simulink library "LIB_TF_G_12_StepControl"  (Simulink 8.6)
settings: Solver=ode45  StartTime=0.0  StopTime=10.0  RelTol=1e-3
PreLoadFcn:
  | if exist('tl_preloadfcn','file'), tl_preloadfcn(gcs,402); end
PostLoadFcn:
  | if exist('tl_postloadfcn','file'), tl_postloadfcn(gcs,402); end
undefined symbols (not defined in the file or in its folder): ddv
libraries: tllib x2
(part 1 of 2)
CloseFcn:
  | if exist('tl_closefcn','file'), tl_closefcn(gcs); end
settings Model: TLRevision=402  Creator=cedric.sauvage  LastModifiedBy=ioan.repede

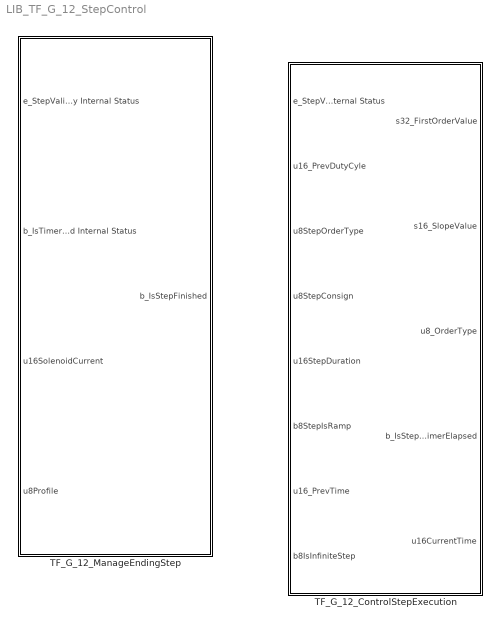
== system LIB_TF_G_12_StepControl ==
  TF_G_12_ControlStepExecution : Subsystem  TreatAsAtomicUnit=on
  TF_G_12_ManageEndingStep : Subsystem  TreatAsAtomicUnit=on

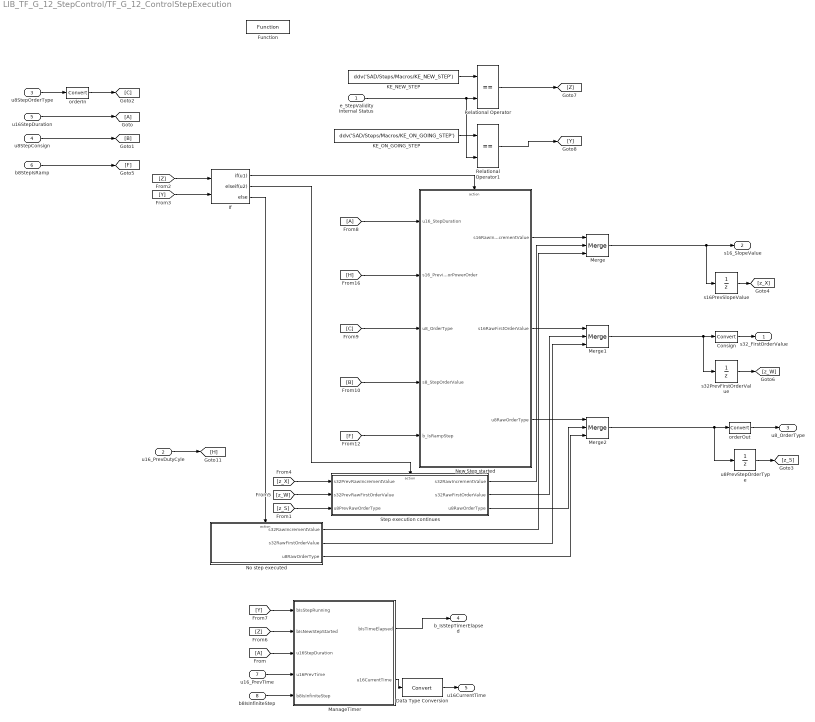
== system LIB_TF_G_12_StepControl/TF_G_12_ControlStepExecution ==
  e_StepValidity Internal Status : Inport
  u16_PrevDutyCyle : Inport  Port=2
  u8StepOrderType : Inport  Port=3
  u8StepConsign : Inport  Port=4
  u16StepDuration : Inport  Port=5
  b8StepIsRamp : Inport  Port=6
  u16_PrevTime : Inport  Port=7
  b8IsInfiniteStep : Inport  Port=8
  Consign : DataTypeConversion  mask(TL_Rescaler){data={'logdata',{'loggingmode',1},'output',{'type','UInt16'},'date',738430.45688642364}}
      settings: DeleteFcn=if exist('delete_tlblock','file')==2,delete_tlblock(gcbh);end  NameChangeFcn=if exist('rename_tlblock','file')==2,rename_tlblock(gcbh);end  OpenFcn=if exist('tl_open_blockdlg','file')==2,tl_open_blockdlg(gcbh);else,open_system(gcbh,'parameter');end
      mask Help: eval(['if exist(''tl_online_help'',''file'') == 2, tl_online_help(''Topic'',''TL_Rescaler''),else, web([''jar:file:///'',matlabroot,''/help/toolbox/simulink/help.jar!/slref/' lower(get_param(gcbh,'Blocktype')) '.html''], ''-helpbrowser''),end'])
      mask Display: plot([-0.1, 1.05, NaN, -0.1, 1.05],[.01, .01, NaN, .99, .99]);
  Data Type Conversion : DataTypeConversion
  Function : tllib/Function  RequirementInfo={'other' '..\..\..\..\Documents and Settings\cedric.sauvage\Desktop\BFE_Design.doc' '@Simulink_requirement_item_16' 'true' 'DSG_BFE_00033' '' } %GIDa_aa7399e7_4aec_40ce_b84e_da620cbb38ff  data={'stepfunctionname','M_ControlStepExecution','stepfunctionclass','STATIC_FCN','codecomment',['[COVERS: DSG_BFE_00033]'],'date',738317.69240863423}  displayString=FUNCTION
  If : If  RequirementInfo={} %GIDa_dfdbd0a4_334d_4bd1_9cca_3fcb5b10a1a1  NumInputs=2  IfExpression=u1  ElseIfExpressions=u2
  KE_NEW_STEP : Constant  Value=ddv('SAD/Steps/Macros/KE_NEW_STEP')  mask(TL_Constant){data={'output',{'variable','SAD/Steps/Macros/KE_NEW_STEP'},'date',738317.69197002309}}
      settings: CopyFcn=if exist('tl_reset_reviewflag','file')==2,tl_reset_reviewflag(gcbh);end  DeleteFcn=if exist('delete_tlblock','file')==2,delete_tlblock(gcbh);end  NameChangeFcn=if exist('rename_tlblock','file')==2,rename_tlblock(gcbh);end  OpenFcn=if exist('tl_open_blockdlg','file')==2,tl_open_blockdlg(gcbh);else,open_system(gcbh,'parameter');end
      mask Help: eval(['if exist(''tl_online_help'',''file'') == 2, tl_online_help(''Topic'',''TL_Constant''),else, web([''jar:file:///'',matlabroot,''/help/toolbox/simulink/help.jar!/slref/' lower(get_param(gcbh,'Blocktype')) '.html''], ''-helpbrowser''),end'])
      mask Display: plot([-0.05, 1.05, NaN, -0.05, 1.05],[.01, .01, NaN, .99, .99])
  KE_ON_GOING_STEP : Constant  Value=ddv('SAD/Steps/Macros/KE_ON_GOING_STEP')  mask(TL_Constant){data={'output',{'variable','SAD/Steps/Macros/KE_ON_GOING_STEP'},'date',738317.69212677085}}
      settings: CopyFcn=if exist('tl_reset_reviewflag','file')==2,tl_reset_reviewflag(gcbh);end  DeleteFcn=if exist('delete_tlblock','file')==2,delete_tlblock(gcbh);end  NameChangeFcn=if exist('rename_tlblock','file')==2,rename_tlblock(gcbh);end  OpenFcn=if exist('tl_open_blockdlg','file')==2,tl_open_blockdlg(gcbh);else,open_system(gcbh,'parameter');end
      mask Help: eval(['if exist(''tl_online_help'',''file'') == 2, tl_online_help(''Topic'',''TL_Constant''),else, web([''jar:file:///'',matlabroot,''/help/toolbox/simulink/help.jar!/slref/' lower(get_param(gcbh,'Blocktype')) '.html''], ''-helpbrowser''),end'])
      mask Display: plot([-0.05, 1.05, NaN, -0.05, 1.05],[.01, .01, NaN, .99, .99])
  ManageTimer : Subsystem  RequirementInfo={} %GIDa_1c6e116c_deb6_4c8b_9c2a_a3ed8f535171  TreatAsAtomicUnit=on
      settings: RTWFcnNameOpts=Use subsystem name
  Merge : Merge  Inputs=3  InitialOutput=0  mask(TL_Merge){data={'output',{'name','s32RawIncrementValue'},'date',735951.66799646989}}
      settings: CopyFcn=if exist('tl_reset_reviewflag','file')==2,tl_reset_reviewflag(gcbh);end  DeleteFcn=if exist('delete_tlblock','file')==2,delete_tlblock(gcbh);end  NameChangeFcn=if exist('rename_tlblock','file')==2,rename_tlblock(gcbh);end  OpenFcn=if exist('tl_open_blockdlg','file')==2,tl_open_blockdlg(gcbh);else,open_system(gcbh,'parameter');end
      mask Help: eval(['if exist(''tl_online_help'',''file'') == 2, tl_online_help(''Topic'',''TL_Merge''),else, web([''jar:file:///'',matlabroot,''/help/toolbox/simulink/help.jar!/slref/' lower(get_param(gcbh,'Blocktype')) '.html''], ''-helpbrowser''),end'])
      mask Display: plot([-0.05, 1.05, NaN, -0.05, 1.05],[.01, .01, NaN, .99, .99])
  Merge1 : Merge  Inputs=3  InitialOutput=0  mask(TL_Merge){data={'output',{'name','s32RawFirstOrderValue'},'date',735951.66799608793}}
      settings: CopyFcn=if exist('tl_reset_reviewflag','file')==2,tl_reset_reviewflag(gcbh);end  DeleteFcn=if exist('delete_tlblock','file')==2,delete_tlblock(gcbh);end  NameChangeFcn=if exist('rename_tlblock','file')==2,rename_tlblock(gcbh);end  OpenFcn=if exist('tl_open_blockdlg','file')==2,tl_open_blockdlg(gcbh);else,open_system(gcbh,'parameter');end
      mask Help: eval(['if exist(''tl_online_help'',''file'') == 2, tl_online_help(''Topic'',''TL_Merge''),else, web([''jar:file:///'',matlabroot,''/help/toolbox/simulink/help.jar!/slref/' lower(get_param(gcbh,'Blocktype')) '.html''], ''-helpbrowser''),end'])
      mask Display: plot([-0.05, 1.05, NaN, -0.05, 1.05],[.01, .01, NaN, .99, .99])
  Merge2 : Merge  RequirementInfo={} %GIDa_81538ec5_5da8_4e36_98a9_b64854f730e2  Inputs=3  InitialOutput=7  mask(TL_Merge){data={'output',{'name','u8RawOrderType'},'date',738370.40050972218}}
      settings: CopyFcn=if exist('tl_reset_reviewflag','file')==2,tl_reset_reviewflag(gcbh);end  DeleteFcn=if exist('delete_tlblock','file')==2,delete_tlblock(gcbh);end  NameChangeFcn=if exist('rename_tlblock','file')==2,rename_tlblock(gcbh);end  OpenFcn=if exist('tl_open_blockdlg','file')==2,tl_open_blockdlg(gcbh);else,open_system(gcbh,'parameter');end
      mask Help: eval(['if exist(''tl_online_help'',''file'') == 2, tl_online_help(''Topic'',''TL_Merge''),else, web([''jar:file:///'',matlabroot,''/help/toolbox/simulink/help.jar!/slref/' lower(get_param(gcbh,'Blocktype')) '.html''], ''-helpbrowser''),end'])
      mask Display: plot([-0.05, 1.05, NaN, -0.05, 1.05],[.01, .01, NaN, .99, .99])
  New Step started : Subsystem  TreatAsAtomicUnit=on
  No step executed : Subsystem  TreatAsAtomicUnit=on
  Relational Operator : RelationalOperator  Operator===  OutDataTypeStr=boolean  mask(TL_RelationalOperator){data={'output',{'name','bIsNewStepStarted'},'date',735951.66796164354}}
      settings: DeleteFcn=if exist('delete_tlblock','file')==2,delete_tlblock(gcbh);end  NameChangeFcn=if exist('rename_tlblock','file')==2,rename_tlblock(gcbh);end  OpenFcn=if exist('tl_open_blockdlg','file')==2,tl_open_blockdlg(gcbh);else,open_system(gcbh,'parameter');end
      mask Help: eval(['if exist(''tl_online_help'',''file'') == 2, tl_online_help(''Topic'',''TL_RelationalOperator''),else, web([''jar:file:///'',matlabroot,''/help/toolbox/simulink/help.jar!/slref/' lower(get_param(gcbh,'Blocktype')) '.html''], ''-helpbrowser''),end'])
      mask Display: plot([-0.05, 1.05, NaN, -0.05, 1.05],[.01, .01, NaN, .99, .99])
  Relational Operator1 : RelationalOperator  Operator===  OutDataTypeStr=boolean  mask(TL_RelationalOperator){data={'date',735951.66796138894}}
      settings: DeleteFcn=if exist('delete_tlblock','file')==2,delete_tlblock(gcbh);end  NameChangeFcn=if exist('rename_tlblock','file')==2,rename_tlblock(gcbh);end  OpenFcn=if exist('tl_open_blockdlg','file')==2,tl_open_blockdlg(gcbh);else,open_system(gcbh,'parameter');end
      mask Help: eval(['if exist(''tl_online_help'',''file'') == 2, tl_online_help(''Topic'',''TL_RelationalOperator''),else, web([''jar:file:///'',matlabroot,''/help/toolbox/simulink/help.jar!/slref/' lower(get_param(gcbh,'Blocktype')) '.html''], ''-helpbrowser''),end'])
      mask Display: plot([-0.05, 1.05, NaN, -0.05, 1.05],[.01, .01, NaN, .99, .99])
  Step execution continues : Subsystem  TreatAsAtomicUnit=on
  orderIn : DataTypeConversion  mask(TL_Rescaler){data={'logdata',{'loggingmode',1},'output',{'type','UInt8'},'date',738370.35603731486}}
      settings: DeleteFcn=if exist('delete_tlblock','file')==2,delete_tlblock(gcbh);end  NameChangeFcn=if exist('rename_tlblock','file')==2,rename_tlblock(gcbh);end  OpenFcn=if exist('tl_open_blockdlg','file')==2,tl_open_blockdlg(gcbh);else,open_system(gcbh,'parameter');end
      mask Help: eval(['if exist(''tl_online_help'',''file'') == 2, tl_online_help(''Topic'',''TL_Rescaler''),else, web([''jar:file:///'',matlabroot,''/help/toolbox/simulink/help.jar!/slref/' lower(get_param(gcbh,'Blocktype')) '.html''], ''-helpbrowser''),end'])
      mask Display: plot([-0.1, 1.05, NaN, -0.1, 1.05],[.01, .01, NaN, .99, .99]);
  orderOut : DataTypeConversion  mask(TL_Rescaler){data={'logdata',{'loggingmode',1},'output',{'type','UInt8'},'date',738370.35619172454}}
      settings: DeleteFcn=if exist('delete_tlblock','file')==2,delete_tlblock(gcbh);end  NameChangeFcn=if exist('rename_tlblock','file')==2,rename_tlblock(gcbh);end  OpenFcn=if exist('tl_open_blockdlg','file')==2,tl_open_blockdlg(gcbh);else,open_system(gcbh,'parameter');end
      mask Help: eval(['if exist(''tl_online_help'',''file'') == 2, tl_online_help(''Topic'',''TL_Rescaler''),else, web([''jar:file:///'',matlabroot,''/help/toolbox/simulink/help.jar!/slref/' lower(get_param(gcbh,'Blocktype')) '.html''], ''-helpbrowser''),end'])
      mask Display: plot([-0.1, 1.05, NaN, -0.1, 1.05],[.01, .01, NaN, .99, .99]);
  s16PrevSlopeValue : UnitDelay  SampleTime=-1  mask(TL_UnitDelay){data={'date',738657.55088192131}}
      settings: CopyFcn=if exist('tl_reset_reviewflag') == 2, tl_reset_reviewflag(gcbh); end  DeleteFcn=if exist('delete_tlblock','file')==2,delete_tlblock(gcbh);end  NameChangeFcn=if exist('rename_tlblock','file')==2,rename_tlblock(gcbh);end  OpenFcn=if exist('tl_open_blockdlg','file')==2,tl_open_blockdlg(gcbh);else,open_system(gcbh,'parameter');end
      mask Help: eval(['if exist(''tl_online_help'',''file'') == 2, tl_online_help(''Topic'',''TL_UnitDelay''),else, web([''jar:file:///'',matlabroot,''/help/toolbox/simulink/help.jar!/slref/' lower(get_param(gcbh,'Blocktype')) '.html''], ''-helpbrowser''),end'])
      mask Display: plot([-0.1, 1.05, NaN, -0.1, 1.05],[.01, .01, NaN, .99, .99]);
  s32PrevFirstOrderValue : UnitDelay  SampleTime=-1  mask(TL_UnitDelay){data={'output',{'type','UInt16'},'state',{'type','UInt16'},'date',738657.55099120375}}
      settings: CopyFcn=if exist('tl_reset_reviewflag') == 2, tl_reset_reviewflag(gcbh); end  DeleteFcn=if exist('delete_tlblock','file')==2,delete_tlblock(gcbh);end  NameChangeFcn=if exist('rename_tlblock','file')==2,rename_tlblock(gcbh);end  OpenFcn=if exist('tl_open_blockdlg','file')==2,tl_open_blockdlg(gcbh);else,open_system(gcbh,'parameter');end
      mask Help: eval(['if exist(''tl_online_help'',''file'') == 2, tl_online_help(''Topic'',''TL_UnitDelay''),else, web([''jar:file:///'',matlabroot,''/help/toolbox/simulink/help.jar!/slref/' lower(get_param(gcbh,'Blocktype')) '.html''], ''-helpbrowser''),end'])
      mask Display: plot([-0.1, 1.05, NaN, -0.1, 1.05],[.01, .01, NaN, .99, .99]);
  u8PrevStepOrderType : UnitDelay  SampleTime=-1  mask(TL_UnitDelay){data={'output',{'type','UInt8'},'state',{'type','UInt8'},'date',738657.45733107638}}
      settings: CopyFcn=if exist('tl_reset_reviewflag') == 2, tl_reset_reviewflag(gcbh); end  DeleteFcn=if exist('delete_tlblock','file')==2,delete_tlblock(gcbh);end  NameChangeFcn=if exist('rename_tlblock','file')==2,rename_tlblock(gcbh);end  OpenFcn=if exist('tl_open_blockdlg','file')==2,tl_open_blockdlg(gcbh);else,open_system(gcbh,'parameter');end
      mask Help: eval(['if exist(''tl_online_help'',''file'') == 2, tl_online_help(''Topic'',''TL_UnitDelay''),else, web([''jar:file:///'',matlabroot,''/help/toolbox/simulink/help.jar!/slref/' lower(get_param(gcbh,'Blocktype')) '.html''], ''-helpbrowser''),end'])
      mask Display: plot([-0.1, 1.05, NaN, -0.1, 1.05],[.01, .01, NaN, .99, .99]);
  s32_FirstOrderValue : Outport
  s16_SlopeValue : Outport  Port=2
  u8_OrderType : Outport  Port=3
  b_IsStepTimerElapsed : Outport  Port=4
  u16CurrentTime : Outport  Port=5
  wires:
  No step executed/3(u8RawOrderType) -> Merge2/3
  Step execution continues/3(u8RawOrderType) -> Merge2/2
  New Step started/3(u8RawOrderType) -> Merge2/1
  u16StepDuration/1 -> [A]
  u8StepOrderType/1 -> orderIn/1
  b8StepIsRamp/1 -> [F]
  ManageTimer/1(bIsTimeElapsed) -> b_IsStepTimerElapsed/1
  [A] -> ManageTimer/3(u16StepDuration)
  e_StepValidity Internal Status/1 -> Relational Operator/2, Relational Operator1/2
  KE_NEW_STEP/1 -> Relational Operator/1
  KE_ON_GOING_STEP/1 -> Relational Operator1/1
  Relational Operator/1 -> [Z]
  Relational Operator1/1 -> [Y]
  [Z] -> If/1
  If/1 -> New Step started/Action
  [Y] -> If/2
  If/2 -> Step execution continues/Action
  If/3 -> No step executed/Action
  New Step started/1(s16RawIncrementValue) -> Merge/1
  New Step started/2(s16RawFirstOrderValue) -> Merge1/1
  Step execution continues/1(s32RawIncrementValue) -> Merge/2
  No step executed/1(s32RawIncrementValue) -> Merge/3
  Step execution continues/2(s32RawFirstOrderValue) -> Merge1/2
  No step executed/2(s32RawFirstOrderValue) -> Merge1/3
  [Z] -> ManageTimer/2(bIsNewStepStarted)
  [Y] -> ManageTimer/1(bIsStepRunning)
  [A] -> New Step started/1(u16_StepDuration)
  [C] -> New Step started/3(u8_OrderType)
  [B] -> New Step started/4(s8_StepOrderValue)
  [F] -> New Step started/5(b_IsRampStep)
  [H] -> New Step started/2(s16_PreviousMotorPowerOrder)
  u16_PrevDutyCyle/1 -> [H]
  Merge2/1 -> u8PrevStepOrderType/1, orderOut/1
  ManageTimer/2(u16CurrentTime) -> Data Type Conversion/1
  u16_PrevTime/1 -> ManageTimer/4(u16PrevTime)
  Data Type Conversion/1 -> u16CurrentTime/1
  orderOut/1 -> u8_OrderType/1
  orderIn/1 -> [C]
  Merge1/1 -> s32PrevFirstOrderValue/1, Consign/1
  u8StepConsign/1 -> [B]
  [z_S] -> Step execution continues/3(u8PrevRawOrderType)
  b8IsInfiniteStep/1 -> ManageTimer/5(b8IsInfiniteStep)
  Consign/1 -> s32_FirstOrderValue/1
  u8PrevStepOrderType/1 -> [z_S]
  Merge/1 -> s16PrevSlopeValue/1, s16_SlopeValue/1
  s16PrevSlopeValue/1 -> [z_X]
  s32PrevFirstOrderValue/1 -> [z_W]
  [z_X] -> Step execution continues/1(s32PrevRawIncrementValue)
  [z_W] -> Step execution continues/2(s32PrevRawFirstOrderValue)

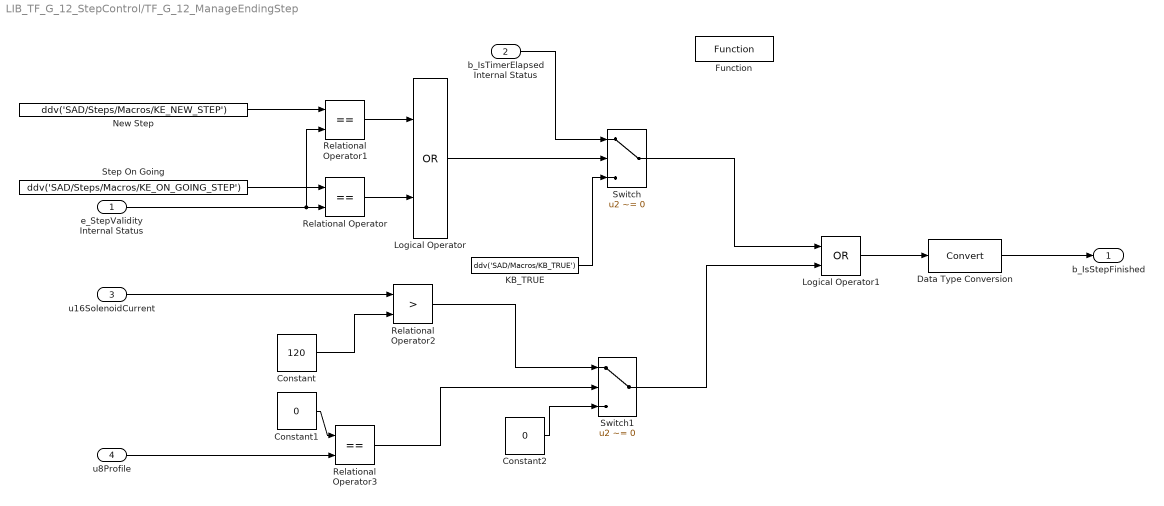
== system LIB_TF_G_12_StepControl/TF_G_12_ManageEndingStep ==
  e_StepValidity Internal Status : Inport
  b_IsTimerElapsed Internal Status : Inport  Port=2
  u16SolenoidCurrent : Inport  Port=3
  u8Profile : Inport  Port=4
  Constant : Constant  Value=120  mask(TL_Constant){data={'date',738645.658251088}}
      settings: CopyFcn=if exist('tl_reset_reviewflag') == 2, tl_reset_reviewflag(gcbh); end  DeleteFcn=if exist('delete_tlblock','file')==2,delete_tlblock(gcbh);end  NameChangeFcn=if exist('rename_tlblock','file')==2,rename_tlblock(gcbh);end  OpenFcn=if exist('tl_open_blockdlg','file')==2,tl_open_blockdlg(gcbh);else,open_system(gcbh,'parameter');end
      mask Help: eval(['if exist(''tl_online_help'',''file'') == 2, tl_online_help(''Topic'',''TL_Constant''),else, web([''jar:file:///'',matlabroot,''/help/toolbox/simulink/help.jar!/slref/' lower(get_param(gcbh,'Blocktype')) '.html''], ''-helpbrowser''),end'])
      mask Display: plot([-0.1, 1.05, NaN, -0.1, 1.05],[.01, .01, NaN, .99, .99]);
  Constant1 : Constant  Value=0  mask(TL_Constant){data={'date',738645.63410811347}}
      settings: CopyFcn=if exist('tl_reset_reviewflag') == 2, tl_reset_reviewflag(gcbh); end  DeleteFcn=if exist('delete_tlblock','file')==2,delete_tlblock(gcbh);end  NameChangeFcn=if exist('rename_tlblock','file')==2,rename_tlblock(gcbh);end  OpenFcn=if exist('tl_open_blockdlg','file')==2,tl_open_blockdlg(gcbh);else,open_system(gcbh,'parameter');end
      mask Help: eval(['if exist(''tl_online_help'',''file'') == 2, tl_online_help(''Topic'',''TL_Constant''),else, web([''jar:file:///'',matlabroot,''/help/toolbox/simulink/help.jar!/slref/' lower(get_param(gcbh,'Blocktype')) '.html''], ''-helpbrowser''),end'])
      mask Display: plot([-0.1, 1.05, NaN, -0.1, 1.05],[.01, .01, NaN, .99, .99]);
  Constant2 : Constant  Value=0  mask(TL_Constant){data={'date',738645.63493682875}}
      settings: CopyFcn=if exist('tl_reset_reviewflag') == 2, tl_reset_reviewflag(gcbh); end  DeleteFcn=if exist('delete_tlblock','file')==2,delete_tlblock(gcbh);end  NameChangeFcn=if exist('rename_tlblock','file')==2,rename_tlblock(gcbh);end  OpenFcn=if exist('tl_open_blockdlg','file')==2,tl_open_blockdlg(gcbh);else,open_system(gcbh,'parameter');end
      mask Help: eval(['if exist(''tl_online_help'',''file'') == 2, tl_online_help(''Topic'',''TL_Constant''),else, web([''jar:file:///'',matlabroot,''/help/toolbox/simulink/help.jar!/slref/' lower(get_param(gcbh,'Blocktype')) '.html''], ''-helpbrowser''),end'])
      mask Display: plot([-0.1, 1.05, NaN, -0.1, 1.05],[.01, .01, NaN, .99, .99]);
  Data Type Conversion : DataTypeConversion
  Function : tllib/Function  RequirementInfo={} %GIDa_9a6d8b05_ba8e_46f3_971b_8d797ff25032  data={'stepfunctionname','M_ManageStepEvents','stepfunctionclass','STATIC_FCN','restartfunctionname','RESTART_ManageStepEvents','initfunctionname','INIT_ManageStepEvents','termfunctionname','TERM_ManageStepEvents','subsystemid','c','date',738317.68422259262}  displayString=FUNCTION
  KB_TRUE : Constant  RequirementInfo={} %GIDa_6933dfa3_0ae3_4e05_b095_5f75714e2f16  Value=ddv('SAD/Macros/KB_TRUE')  OutDataTypeStr=boolean  mask(TL_Constant){data={'output',{'variable','SAD/Macros/KB_TRUE'},'date',738317.69141375006}}
      settings: CopyFcn=if exist('tl_reset_reviewflag','file')==2,tl_reset_reviewflag(gcbh);end  DeleteFcn=if exist('delete_tlblock','file')==2,delete_tlblock(gcbh);end  NameChangeFcn=if exist('rename_tlblock','file')==2,rename_tlblock(gcbh);end  OpenFcn=if exist('tl_open_blockdlg','file')==2,tl_open_blockdlg(gcbh);else,open_system(gcbh,'parameter');end
      mask Help: eval(['if exist(''tl_online_help'',''file'') == 2, tl_online_help(''Topic'',''TL_Constant''),else, web([''jar:file:///'',matlabroot,''/help/toolbox/simulink/help.jar!/slref/' lower(get_param(gcbh,'Blocktype')) '.html''], ''-helpbrowser''),end'])
      mask Display: plot([-0.05, 1.05, NaN, -0.05, 1.05],[.01, .01, NaN, .99, .99])
  Logical Operator : Logic  Operator=OR  AllPortsSameDT=off  OutDataTypeStr=boolean  mask(TL_LogicalOperator){data={'output',{'name','bIsStepExecutionOnGoing'},'date',735951.66848681716}}
      settings: DeleteFcn=if exist('delete_tlblock','file')==2,delete_tlblock(gcbh);end  NameChangeFcn=if exist('rename_tlblock','file')==2,rename_tlblock(gcbh);end  OpenFcn=if exist('tl_open_blockdlg','file')==2,tl_open_blockdlg(gcbh);else,open_system(gcbh,'parameter');end
      mask Help: eval(['if exist(''tl_online_help'',''file'') == 2, tl_online_help(''Topic'',''TL_LogicalOperator''),else, web([''jar:file:///'',matlabroot,''/help/toolbox/simulink/help.jar!/slref/' lower(get_param(gcbh,'Blocktype')) '.html''], ''-helpbrowser''),end'])
      mask Display: plot([-0.05, 1.05, NaN, -0.05, 1.05],[.01, .01, NaN, .99, .99])
  Logical Operator1 : Logic  Operator=OR  AllPortsSameDT=off  OutDataTypeStr=boolean  mask(TL_LogicalOperator){data={'date',738645.5888651273}}
      settings: DeleteFcn=if exist('delete_tlblock','file')==2,delete_tlblock(gcbh);end  NameChangeFcn=if exist('rename_tlblock','file')==2,rename_tlblock(gcbh);end  OpenFcn=if exist('tl_open_blockdlg','file')==2,tl_open_blockdlg(gcbh);else,open_system(gcbh,'parameter');end
      mask Help: eval(['if exist(''tl_online_help'',''file'') == 2, tl_online_help(''Topic'',''TL_LogicalOperator''),else, web([''jar:file:///'',matlabroot,''/help/toolbox/simulink/help.jar!/slref/' lower(get_param(gcbh,'Blocktype')) '.html''], ''-helpbrowser''),end'])
      mask Display: plot([-0.1, 1.05, NaN, -0.1, 1.05],[.01, .01, NaN, .99, .99]);
  New Step : Constant  Value=ddv('SAD/Steps/Macros/KE_NEW_STEP')  mask(TL_Constant){data={'output',{'variable','SAD/Steps/Macros/KE_NEW_STEP'},'date',738317.69161768514}}
      settings: CopyFcn=if exist('tl_reset_reviewflag','file')==2,tl_reset_reviewflag(gcbh);end  DeleteFcn=if exist('delete_tlblock','file')==2,delete_tlblock(gcbh);end  NameChangeFcn=if exist('rename_tlblock','file')==2,rename_tlblock(gcbh);end  OpenFcn=if exist('tl_open_blockdlg','file')==2,tl_open_blockdlg(gcbh);else,open_system(gcbh,'parameter');end
      mask Help: eval(['if exist(''tl_online_help'',''file'') == 2, tl_online_help(''Topic'',''TL_Constant''),else, web([''jar:file:///'',matlabroot,''/help/toolbox/simulink/help.jar!/slref/' lower(get_param(gcbh,'Blocktype')) '.html''], ''-helpbrowser''),end'])
      mask Display: plot([-0.05, 1.05, NaN, -0.05, 1.05],[.01, .01, NaN, .99, .99])
  Relational Operator : RelationalOperator  Operator===  OutDataTypeStr=boolean  mask(TL_RelationalOperator){data={'date',735951.66848545137}}
      settings: DeleteFcn=if exist('delete_tlblock','file')==2,delete_tlblock(gcbh);end  NameChangeFcn=if exist('rename_tlblock','file')==2,rename_tlblock(gcbh);end  OpenFcn=if exist('tl_open_blockdlg','file')==2,tl_open_blockdlg(gcbh);else,open_system(gcbh,'parameter');end
      mask Help: eval(['if exist(''tl_online_help'',''file'') == 2, tl_online_help(''Topic'',''TL_RelationalOperator''),else, web([''jar:file:///'',matlabroot,''/help/toolbox/simulink/help.jar!/slref/' lower(get_param(gcbh,'Blocktype')) '.html''], ''-helpbrowser''),end'])
      mask Display: plot([-0.05, 1.05, NaN, -0.05, 1.05],[.01, .01, NaN, .99, .99])
  Relational Operator1 : RelationalOperator  Operator===  OutDataTypeStr=boolean  mask(TL_RelationalOperator){data={'date',735951.6684852083}}
      settings: DeleteFcn=if exist('delete_tlblock','file')==2,delete_tlblock(gcbh);end  NameChangeFcn=if exist('rename_tlblock','file')==2,rename_tlblock(gcbh);end  OpenFcn=if exist('tl_open_blockdlg','file')==2,tl_open_blockdlg(gcbh);else,open_system(gcbh,'parameter');end
      mask Help: eval(['if exist(''tl_online_help'',''file'') == 2, tl_online_help(''Topic'',''TL_RelationalOperator''),else, web([''jar:file:///'',matlabroot,''/help/toolbox/simulink/help.jar!/slref/' lower(get_param(gcbh,'Blocktype')) '.html''], ''-helpbrowser''),end'])
      mask Display: plot([-0.05, 1.05, NaN, -0.05, 1.05],[.01, .01, NaN, .99, .99])
  Relational Operator2 : RelationalOperator  Operator=>  OutDataTypeStr=boolean  mask(TL_RelationalOperator){data={'date',738645.57967488421}}
      settings: DeleteFcn=if exist('delete_tlblock','file')==2,delete_tlblock(gcbh);end  NameChangeFcn=if exist('rename_tlblock','file')==2,rename_tlblock(gcbh);end  OpenFcn=if exist('tl_open_blockdlg','file')==2,tl_open_blockdlg(gcbh);else,open_system(gcbh,'parameter');end
      mask Help: eval(['if exist(''tl_online_help'',''file'') == 2, tl_online_help(''Topic'',''TL_RelationalOperator''),else, web([''jar:file:///'',matlabroot,''/help/toolbox/simulink/help.jar!/slref/' lower(get_param(gcbh,'Blocktype')) '.html''], ''-helpbrowser''),end'])
      mask Display: plot([-0.1, 1.05, NaN, -0.1, 1.05],[.01, .01, NaN, .99, .99]);
  Relational Operator3 : RelationalOperator  Operator===  OutDataTypeStr=boolean  mask(TL_RelationalOperator){data={'date',738645.63418839115}}
      settings: DeleteFcn=if exist('delete_tlblock','file')==2,delete_tlblock(gcbh);end  NameChangeFcn=if exist('rename_tlblock','file')==2,rename_tlblock(gcbh);end  OpenFcn=if exist('tl_open_blockdlg','file')==2,tl_open_blockdlg(gcbh);else,open_system(gcbh,'parameter');end
      mask Help: eval(['if exist(''tl_online_help'',''file'') == 2, tl_online_help(''Topic'',''TL_RelationalOperator''),else, web([''jar:file:///'',matlabroot,''/help/toolbox/simulink/help.jar!/slref/' lower(get_param(gcbh,'Blocktype')) '.html''], ''-helpbrowser''),end'])
      mask Display: plot([-0.1, 1.05, NaN, -0.1, 1.05],[.01, .01, NaN, .99, .99]);
  Step On Going : Constant  Value=ddv('SAD/Steps/Macros/KE_ON_GOING_STEP')  mask(TL_Constant){data={'output',{'variable','SAD/Steps/Macros/KE_ON_GOING_STEP'},'date',738317.69126152783}}
      settings: CopyFcn=if exist('tl_reset_reviewflag','file')==2,tl_reset_reviewflag(gcbh);end  DeleteFcn=if exist('delete_tlblock','file')==2,delete_tlblock(gcbh);end  NameChangeFcn=if exist('rename_tlblock','file')==2,rename_tlblock(gcbh);end  OpenFcn=if exist('tl_open_blockdlg','file')==2,tl_open_blockdlg(gcbh);else,open_system(gcbh,'parameter');end
      mask Help: eval(['if exist(''tl_online_help'',''file'') == 2, tl_online_help(''Topic'',''TL_Constant''),else, web([''jar:file:///'',matlabroot,''/help/toolbox/simulink/help.jar!/slref/' lower(get_param(gcbh,'Blocktype')) '.html''], ''-helpbrowser''),end'])
      mask Display: plot([-0.05, 1.05, NaN, -0.05, 1.05],[.01, .01, NaN, .99, .99])
  Switch : Switch  Criteria=u2 ~= 0  mask(TL_Switch){data={'output',{'type','Bool'},'date',738645.58603942127}}
      settings: CopyFcn=if exist('tl_reset_reviewflag') == 2, tl_reset_reviewflag(gcbh); end  DeleteFcn=if exist('delete_tlblock','file')==2,delete_tlblock(gcbh);end  NameChangeFcn=if exist('rename_tlblock','file')==2,rename_tlblock(gcbh);end  OpenFcn=if exist('tl_open_blockdlg','file')==2,tl_open_blockdlg(gcbh);else,open_system(gcbh,'parameter');end
      mask Help: eval(['if exist(''tl_online_help'',''file'') == 2, tl_online_help(''Topic'',''TL_Switch''),else, web([''jar:file:///'',matlabroot,''/help/toolbox/simulink/help.jar!/slref/' lower(get_param(gcbh,'Blocktype')) '.html''], ''-helpbrowser''),end'])
      mask Display: plot([-0.1, 1.05, NaN, -0.1, 1.05],[.01, .01, NaN, .99, .99]);
  Switch1 : Switch  Criteria=u2 ~= 0  mask(TL_Switch){data={'output',{'type','Bool'},'date',738645.63458362268}}
      settings: CopyFcn=if exist('tl_reset_reviewflag') == 2, tl_reset_reviewflag(gcbh); end  DeleteFcn=if exist('delete_tlblock','file')==2,delete_tlblock(gcbh);end  NameChangeFcn=if exist('rename_tlblock','file')==2,rename_tlblock(gcbh);end  OpenFcn=if exist('tl_open_blockdlg','file')==2,tl_open_blockdlg(gcbh);else,open_system(gcbh,'parameter');end
      mask Help: eval(['if exist(''tl_online_help'',''file'') == 2, tl_online_help(''Topic'',''TL_Switch''),else, web([''jar:file:///'',matlabroot,''/help/toolbox/simulink/help.jar!/slref/' lower(get_param(gcbh,'Blocktype')) '.html''], ''-helpbrowser''),end'])
      mask Display: plot([-0.1, 1.05, NaN, -0.1, 1.05],[.01, .01, NaN, .99, .99]);
  b_IsStepFinished : Outport
  wires:
  b_IsTimerElapsed Internal Status/1 -> Switch/1
  Relational Operator/1 -> Logical Operator/2
  Relational Operator1/1 -> Logical Operator/1
  e_StepValidity Internal Status/1 -> Relational Operator/2, Relational Operator1/2
  New Step/1 -> Relational Operator1/1
  Step On Going/1 -> Relational Operator/1
  Logical Operator/1 -> Switch/2
  KB_TRUE/1 -> Switch/3
  u16SolenoidCurrent/1 -> Relational Operator2/1
  Constant/1 -> Relational Operator2/2
  Switch/1 -> Logical Operator1/1
  Logical Operator1/1 -> Data Type Conversion/1
  Data Type Conversion/1 -> b_IsStepFinished/1
  Constant1/1 -> Relational Operator3/1
  u8Profile/1 -> Relational Operator3/2
  Relational Operator3/1 -> Switch1/2
  Relational Operator2/1 -> Switch1/1
  Switch1/1 -> Logical Operator1/2
  Constant2/1 -> Switch1/3

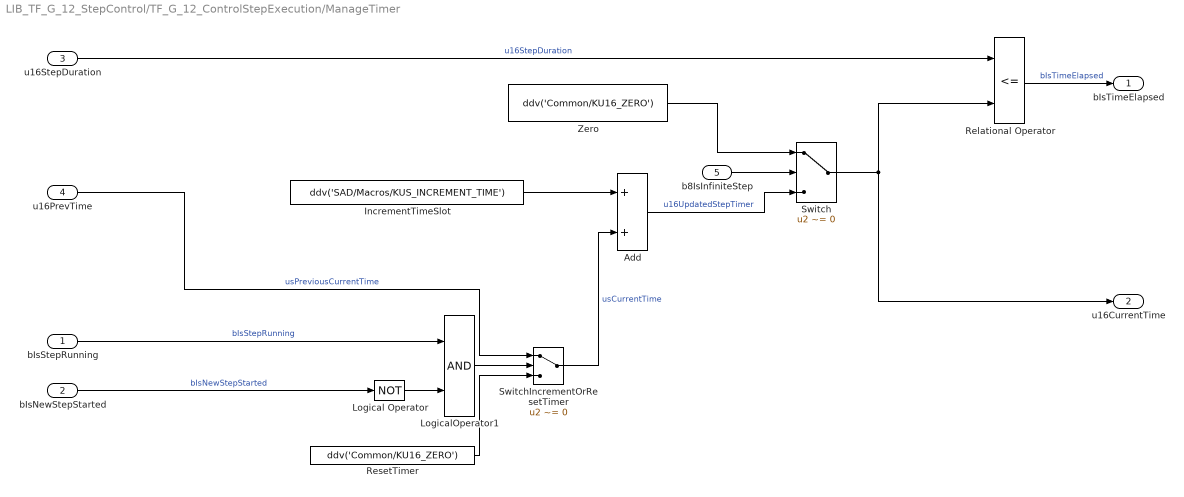
== system LIB_TF_G_12_StepControl/TF_G_12_ControlStepExecution/ManageTimer ==
  bIsStepRunning : Inport  RequirementInfo={} %GIDa_8099bea4_e8c1_4692_a6f9_d176147f505d
  bIsNewStepStarted : Inport  RequirementInfo={} %GIDa_5064309f_314f_43a7_8546_a3acea29a31d  Port=2
  u16StepDuration : Inport  RequirementInfo={} %GIDa_e2682689_4f53_4bd0_88ce_17de940b29c4  Port=3
  u16PrevTime : Inport  RequirementInfo={} %GIDa_e2682689_4f53_4bd0_88ce_17de940b29c4  Port=4
  b8IsInfiniteStep : Inport  RequirementInfo={} %GIDa_e2682689_4f53_4bd0_88ce_17de940b29c4  Port=5
  Add : Sum  RequirementInfo={} %GIDa_29793857_171b_4407_b062_784dd89fa0d8  OutDataTypeStr=uint16  SaturateOnIntegerOverflow=on  mask(TL_Sum){data={'output',{'name','u16UpdatedStepTimer','type','UInt16','checkmin',1,'checkmax',1},'autoscaling',{'mode',2},'date',735951.66800328705}}
      settings: AttributesFormatString=Saturation: %<SaturateOnIntegerOverflow>  CopyFcn=if exist('tl_reset_reviewflag','file')==2,tl_reset_reviewflag(gcbh);end  DeleteFcn=if exist('delete_tlblock','file')==2,delete_tlblock(gcbh);end  NameChangeFcn=if exist('rename_tlblock','file')==2,rename_tlblock(gcbh);end  OpenFcn=if exist('tl_open_blockdlg','file')==2,tl_open_blockdlg(gcbh);else,open_system(gcbh,'parameter');end
      mask Help: eval(['if exist(''tl_online_help'',''file'') == 2, tl_online_help(''Topic'',''TL_Sum''),else, web([''jar:file:///'',matlabroot,''/help/toolbox/simulink/help.jar!/slref/' lower(get_param(gcbh,'Blocktype')) '.html''], ''-helpbrowser''),end'])
      mask Display: plot([-0.05, 1.05, NaN, -0.05, 1.05],[.01, .01, NaN, .99, .99])
  IncrementTimeSlot : Constant  RequirementInfo={} %GIDa_30227bc5_f72d_4077_9beb_be89df347bf6  Value=ddv('SAD/Macros/KUS_INCREMENT_TIME')  OutDataTypeStr=uint16  mask(TL_Constant){data={'output',{'variable','SAD/Macros/KUS_INCREMENT_TIME'},'date',738321.64903990738}}
      settings: CopyFcn=if exist('tl_reset_reviewflag','file')==2,tl_reset_reviewflag(gcbh);end  DeleteFcn=if exist('delete_tlblock','file')==2,delete_tlblock(gcbh);end  NameChangeFcn=if exist('rename_tlblock','file')==2,rename_tlblock(gcbh);end  OpenFcn=if exist('tl_open_blockdlg','file')==2,tl_open_blockdlg(gcbh);else,open_system(gcbh,'parameter');end
      mask Help: eval(['if exist(''tl_online_help'',''file'') == 2, tl_online_help(''Topic'',''TL_Constant''),else, web([''jar:file:///'',matlabroot,''/help/toolbox/simulink/help.jar!/slref/' lower(get_param(gcbh,'Blocktype')) '.html''], ''-helpbrowser''),end'])
      mask Display: plot([-0.05, 1.05, NaN, -0.05, 1.05],[.01, .01, NaN, .99, .99])
  Logical Operator : Logic  RequirementInfo={} %GIDa_a1686c55_b017_4ac8_bcb6_4b0a82067be0  Operator=NOT  Inputs=1  AllPortsSameDT=off  OutDataTypeStr=boolean  mask(TL_LogicalOperator){data={'date',735951.66800087958}}
      settings: DeleteFcn=if exist('delete_tlblock','file')==2,delete_tlblock(gcbh);end  NameChangeFcn=if exist('rename_tlblock','file')==2,rename_tlblock(gcbh);end  OpenFcn=if exist('tl_open_blockdlg','file')==2,tl_open_blockdlg(gcbh);else,open_system(gcbh,'parameter');end
      mask Help: eval(['if exist(''tl_online_help'',''file'') == 2, tl_online_help(''Topic'',''TL_LogicalOperator''),else, web([''jar:file:///'',matlabroot,''/help/toolbox/simulink/help.jar!/slref/' lower(get_param(gcbh,'Blocktype')) '.html''], ''-helpbrowser''),end'])
      mask Display: plot([-0.05, 1.05, NaN, -0.05, 1.05],[.01, .01, NaN, .99, .99])
  LogicalOperator1 : Logic  RequirementInfo={} %GIDa_4f8d19d4_46ad_40ac_a08b_006477df76af  AllPortsSameDT=off  OutDataTypeStr=boolean  mask(TL_LogicalOperator){data={'date',735951.66800062498}}
      settings: DeleteFcn=if exist('delete_tlblock','file')==2,delete_tlblock(gcbh);end  NameChangeFcn=if exist('rename_tlblock','file')==2,rename_tlblock(gcbh);end  OpenFcn=if exist('tl_open_blockdlg','file')==2,tl_open_blockdlg(gcbh);else,open_system(gcbh,'parameter');end
      mask Help: eval(['if exist(''tl_online_help'',''file'') == 2, tl_online_help(''Topic'',''TL_LogicalOperator''),else, web([''jar:file:///'',matlabroot,''/help/toolbox/simulink/help.jar!/slref/' lower(get_param(gcbh,'Blocktype')) '.html''], ''-helpbrowser''),end'])
      mask Display: plot([-0.05, 1.05, NaN, -0.05, 1.05],[.01, .01, NaN, .99, .99])
  Relational Operator : RelationalOperator  RequirementInfo={} %GIDa_885072fa_b492_4d65_aaa4_c1413b1c79d5  Operator=<=  OutDataTypeStr=boolean  mask(TL_RelationalOperator){data={'output',{'name','bIsTimerElapsed'},'date',735951.66799986106}}
      settings: DeleteFcn=if exist('delete_tlblock','file')==2,delete_tlblock(gcbh);end  NameChangeFcn=if exist('rename_tlblock','file')==2,rename_tlblock(gcbh);end  OpenFcn=if exist('tl_open_blockdlg','file')==2,tl_open_blockdlg(gcbh);else,open_system(gcbh,'parameter');end
      mask Help: eval(['if exist(''tl_online_help'',''file'') == 2, tl_online_help(''Topic'',''TL_RelationalOperator''),else, web([''jar:file:///'',matlabroot,''/help/toolbox/simulink/help.jar!/slref/' lower(get_param(gcbh,'Blocktype')) '.html''], ''-helpbrowser''),end'])
      mask Display: plot([-0.05, 1.05, NaN, -0.05, 1.05],[.01, .01, NaN, .99, .99])
  ResetTimer : Constant  RequirementInfo={} %GIDa_d400d14c_fedd_468a_9d55_b734797d539d  Value=ddv('Common/KU16_ZERO')  OutDataTypeStr=uint16  mask(TL_Constant){data={'output',{'variable','Common/KU16_ZERO'},'date',735951.66799936339}}
      settings: CopyFcn=if exist('tl_reset_reviewflag','file')==2,tl_reset_reviewflag(gcbh);end  DeleteFcn=if exist('delete_tlblock','file')==2,delete_tlblock(gcbh);end  NameChangeFcn=if exist('rename_tlblock','file')==2,rename_tlblock(gcbh);end  OpenFcn=if exist('tl_open_blockdlg','file')==2,tl_open_blockdlg(gcbh);else,open_system(gcbh,'parameter');end
      mask Help: eval(['if exist(''tl_online_help'',''file'') == 2, tl_online_help(''Topic'',''TL_Constant''),else, web([''jar:file:///'',matlabroot,''/help/toolbox/simulink/help.jar!/slref/' lower(get_param(gcbh,'Blocktype')) '.html''], ''-helpbrowser''),end'])
      mask Display: plot([-0.05, 1.05, NaN, -0.05, 1.05],[.01, .01, NaN, .99, .99])
  Switch : Switch  Criteria=u2 ~= 0  mask(TL_Switch){data={'output',{'type','UInt16'},'date',738373.37235883099}}
      settings: CopyFcn=if exist('tl_reset_reviewflag') == 2, tl_reset_reviewflag(gcbh); end  DeleteFcn=if exist('delete_tlblock','file')==2,delete_tlblock(gcbh);end  NameChangeFcn=if exist('rename_tlblock','file')==2,rename_tlblock(gcbh);end  OpenFcn=if exist('tl_open_blockdlg','file')==2,tl_open_blockdlg(gcbh);else,open_system(gcbh,'parameter');end
      mask Help: eval(['if exist(''tl_online_help'',''file'') == 2, tl_online_help(''Topic'',''TL_Switch''),else, web([''jar:file:///'',matlabroot,''/help/toolbox/simulink/help.jar!/slref/' lower(get_param(gcbh,'Blocktype')) '.html''], ''-helpbrowser''),end'])
      mask Display: plot([-0.1, 1.05, NaN, -0.1, 1.05],[.01, .01, NaN, .99, .99]);
  SwitchIncrementOrResetTimer : Switch  RequirementInfo={} %GIDa_25344fa8_8921_4960_a2d3_faa64437b123  Criteria=u2 ~= 0  OutDataTypeStr=uint16  SaturateOnIntegerOverflow=on  mask(TL_Switch){data={'output',{'name','u16TimerOrigin','type','UInt16','checkmin',1,'checkmax',1},'autoscaling',{'mode',2},'date',735951.66799805558}}
      settings: CopyFcn=if exist('tl_reset_reviewflag','file')==2,tl_reset_reviewflag(gcbh);end  DeleteFcn=if exist('delete_tlblock','file')==2,delete_tlblock(gcbh);end  NameChangeFcn=if exist('rename_tlblock','file')==2,rename_tlblock(gcbh);end  OpenFcn=if exist('tl_open_blockdlg','file')==2,tl_open_blockdlg(gcbh);else,open_system(gcbh,'parameter');end
      mask Help: eval(['if exist(''tl_online_help'',''file'') == 2, tl_online_help(''Topic'',''TL_Switch''),else, web([''jar:file:///'',matlabroot,''/help/toolbox/simulink/help.jar!/slref/' lower(get_param(gcbh,'Blocktype')) '.html''], ''-helpbrowser''),end'])
      mask Display: plot([-0.05, 1.05, NaN, -0.05, 1.05],[.01, .01, NaN, .99, .99])
  Zero : Constant  Value=ddv('Common/KU16_ZERO')  mask(TL_Constant){data={'output',{'variable','Common/KU16_ZERO'},'date',738373.37323211809}}
      settings: CopyFcn=if exist('tl_reset_reviewflag') == 2, tl_reset_reviewflag(gcbh); end  DeleteFcn=if exist('delete_tlblock','file')==2,delete_tlblock(gcbh);end  NameChangeFcn=if exist('rename_tlblock','file')==2,rename_tlblock(gcbh);end  OpenFcn=if exist('tl_open_blockdlg','file')==2,tl_open_blockdlg(gcbh);else,open_system(gcbh,'parameter');end
      mask Help: eval(['if exist(''tl_online_help'',''file'') == 2, tl_online_help(''Topic'',''TL_Constant''),else, web([''jar:file:///'',matlabroot,''/help/toolbox/simulink/help.jar!/slref/' lower(get_param(gcbh,'Blocktype')) '.html''], ''-helpbrowser''),end'])
      mask Display: plot([-0.1, 1.05, NaN, -0.1, 1.05],[.01, .01, NaN, .99, .99]);
  bIsTimeElapsed : Outport  RequirementInfo={} %GIDa_70338377_5d6f_48f6_ad20_40eecd5f4ea6
  u16CurrentTime : Outport  RequirementInfo={} %GIDa_89bbad4f_06a6_4895_9511_fce3ce958955  Port=2
  wires:
  u16PrevTime/1 -> SwitchIncrementOrResetTimer/1  "usPreviousCurrentTime"
  SwitchIncrementOrResetTimer/1 -> Add/2  "usCurrentTime"
  IncrementTimeSlot/1 -> Add/1
  bIsNewStepStarted/1 -> Logical Operator/1  "bIsNewStepStarted"
  bIsStepRunning/1 -> LogicalOperator1/1  "bIsStepRunning"
  LogicalOperator1/1 -> SwitchIncrementOrResetTimer/2
  Relational Operator/1 -> bIsTimeElapsed/1  "bIsTimeElapsed"
  u16StepDuration/1 -> Relational Operator/1  "u16StepDuration"
  ResetTimer/1 -> SwitchIncrementOrResetTimer/3
  Logical Operator/1 -> LogicalOperator1/2
  b8IsInfiniteStep/1 -> Switch/2
  Add/1 -> Switch/3  "u16UpdatedStepTimer"
  Switch/1 -> Relational Operator/2, u16CurrentTime/1
  Zero/1 -> Switch/1

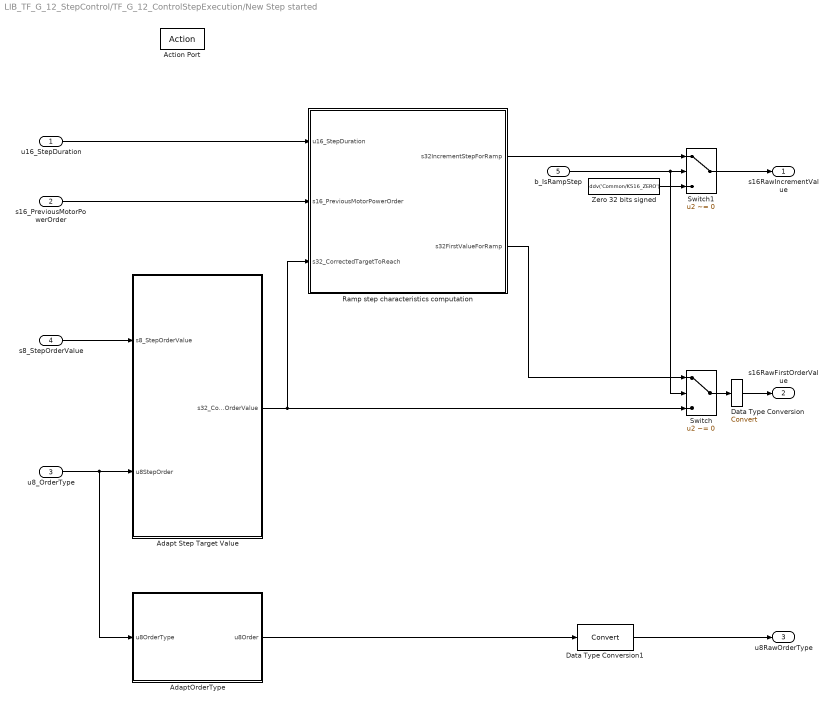
== system LIB_TF_G_12_StepControl/TF_G_12_ControlStepExecution/New Step started ==
  u16_StepDuration : Inport
  s16_PreviousMotorPowerOrder : Inport  Port=2
  u8_OrderType : Inport  Port=3
  s8_StepOrderValue : Inport  Port=4
  b_IsRampStep : Inport  Port=5
  Action Port : ActionPort
  Adapt Step Target Value : Subsystem  TreatAsAtomicUnit=on
  AdaptOrderType : Subsystem  RequirementInfo={} %GIDa_13dc65f5_0a95_4e88_a7b6_c4733fe3f649  TreatAsAtomicUnit=on
  Data Type Conversion : DataTypeConversion
  Data Type Conversion1 : DataTypeConversion
  Ramp step characteristics computation : Subsystem  TreatAsAtomicUnit=on
  Switch : Switch  Criteria=u2 ~= 0  OutDataTypeStr=int32  mask(TL_Switch){data={'output',{'type','UInt16'},'date',738370.66682802083}}
      settings: CopyFcn=if exist('tl_reset_reviewflag','file')==2,tl_reset_reviewflag(gcbh);end  DeleteFcn=if exist('delete_tlblock','file')==2,delete_tlblock(gcbh);end  NameChangeFcn=if exist('rename_tlblock','file')==2,rename_tlblock(gcbh);end  OpenFcn=if exist('tl_open_blockdlg','file')==2,tl_open_blockdlg(gcbh);else,open_system(gcbh,'parameter');end
      mask Help: eval(['if exist(''tl_online_help'',''file'') == 2, tl_online_help(''Topic'',''TL_Switch''),else, web([''jar:file:///'',matlabroot,''/help/toolbox/simulink/help.jar!/slref/' lower(get_param(gcbh,'Blocktype')) '.html''], ''-helpbrowser''),end'])
      mask Display: plot([-0.05, 1.05, NaN, -0.05, 1.05],[.01, .01, NaN, .99, .99])
  Switch1 : Switch  Criteria=u2 ~= 0  mask(TL_Switch){data={'date',738370.61609614582}}
      settings: CopyFcn=if exist('tl_reset_reviewflag','file')==2,tl_reset_reviewflag(gcbh);end  DeleteFcn=if exist('delete_tlblock','file')==2,delete_tlblock(gcbh);end  NameChangeFcn=if exist('rename_tlblock','file')==2,rename_tlblock(gcbh);end  OpenFcn=if exist('tl_open_blockdlg','file')==2,tl_open_blockdlg(gcbh);else,open_system(gcbh,'parameter');end
      mask Help: eval(['if exist(''tl_online_help'',''file'') == 2, tl_online_help(''Topic'',''TL_Switch''),else, web([''jar:file:///'',matlabroot,''/help/toolbox/simulink/help.jar!/slref/' lower(get_param(gcbh,'Blocktype')) '.html''], ''-helpbrowser''),end'])
      mask Display: plot([-0.05, 1.05, NaN, -0.05, 1.05],[.01, .01, NaN, .99, .99])
  Zero 32 bits signed : Constant  Value=ddv('Common/KS16_ZERO')  mask(TL_Constant){data={'output',{'variable','Common/KS16_ZERO'},'date',738322.37265452545}}
      settings: CopyFcn=if exist('tl_reset_reviewflag','file')==2,tl_reset_reviewflag(gcbh);end  DeleteFcn=if exist('delete_tlblock','file')==2,delete_tlblock(gcbh);end  NameChangeFcn=if exist('rename_tlblock','file')==2,rename_tlblock(gcbh);end  OpenFcn=if exist('tl_open_blockdlg','file')==2,tl_open_blockdlg(gcbh);else,open_system(gcbh,'parameter');end
      mask Help: eval(['if exist(''tl_online_help'',''file'') == 2, tl_online_help(''Topic'',''TL_Constant''),else, web([''jar:file:///'',matlabroot,''/help/toolbox/simulink/help.jar!/slref/' lower(get_param(gcbh,'Blocktype')) '.html''], ''-helpbrowser''),end'])
      mask Display: plot([-0.05, 1.05, NaN, -0.05, 1.05],[.01, .01, NaN, .99, .99])
  s16RawIncrementValue : Outport  InitialOutput=0
  s16RawFirstOrderValue : Outport  Port=2  InitialOutput=0
  u8RawOrderType : Outport  Port=3  InitialOutput=7
  wires:
  AdaptOrderType/1(u8Order) -> Data Type Conversion1/1
  u8_OrderType/1 -> AdaptOrderType/1(u8OrderType), Adapt Step Target Value/2(u8StepOrder)
  s8_StepOrderValue/1 -> Adapt Step Target Value/1(s8_StepOrderValue)
  Switch1/1 -> s16RawIncrementValue/1
  Switch/1 -> Data Type Conversion/1
  b_IsRampStep/1 -> Switch1/2, Switch/2
  Zero 32 bits signed/1 -> Switch1/3
  Ramp step characteristics computation/1(s32IncrementStepForRamp) -> Switch1/1
  Ramp step characteristics computation/2(s32FirstValueForRamp) -> Switch/1
  s16_PreviousMotorPowerOrder/1 -> Ramp step characteristics computation/2(s16_PreviousMotorPowerOrder)
  Data Type Conversion/1 -> s16RawFirstOrderValue/1
  u16_StepDuration/1 -> Ramp step characteristics computation/1(u16_StepDuration)
  Data Type Conversion1/1 -> u8RawOrderType/1
  Adapt Step Target Value/1(s32_CorrectedOrderValue) -> Ramp step characteristics computation/3(s32_CorrectedTargetToReach), Switch/3

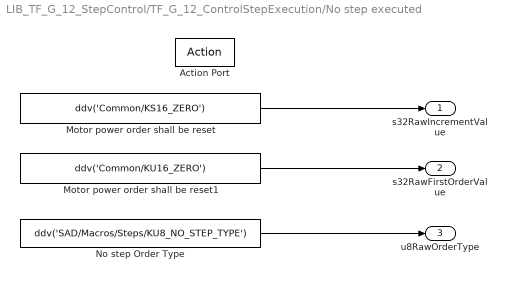
== system LIB_TF_G_12_StepControl/TF_G_12_ControlStepExecution/No step executed ==
  Action Port : ActionPort
  Motor power order shall be reset : Constant  Value=ddv('Common/KS16_ZERO')  mask(TL_Constant){data={'output',{'variable','Common/KS16_ZERO'},'date',738370.61657325237}}
      settings: CopyFcn=if exist('tl_reset_reviewflag','file')==2,tl_reset_reviewflag(gcbh);end  DeleteFcn=if exist('delete_tlblock','file')==2,delete_tlblock(gcbh);end  NameChangeFcn=if exist('rename_tlblock','file')==2,rename_tlblock(gcbh);end  OpenFcn=if exist('tl_open_blockdlg','file')==2,tl_open_blockdlg(gcbh);else,open_system(gcbh,'parameter');end
      mask Help: eval(['if exist(''tl_online_help'',''file'') == 2, tl_online_help(''Topic'',''TL_Constant''),else, web([''jar:file:///'',matlabroot,''/help/toolbox/simulink/help.jar!/slref/' lower(get_param(gcbh,'Blocktype')) '.html''], ''-helpbrowser''),end'])
      mask Display: plot([-0.05, 1.05, NaN, -0.05, 1.05],[.01, .01, NaN, .99, .99])
  Motor power order shall be reset1 : Constant  Value=ddv('Common/KU16_ZERO')  mask(TL_Constant){data={'output',{'variable','Common/KU16_ZERO'},'date',738370.684536007}}
      settings: CopyFcn=if exist('tl_reset_reviewflag','file')==2,tl_reset_reviewflag(gcbh);end  DeleteFcn=if exist('delete_tlblock','file')==2,delete_tlblock(gcbh);end  NameChangeFcn=if exist('rename_tlblock','file')==2,rename_tlblock(gcbh);end  OpenFcn=if exist('tl_open_blockdlg','file')==2,tl_open_blockdlg(gcbh);else,open_system(gcbh,'parameter');end
      mask Help: eval(['if exist(''tl_online_help'',''file'') == 2, tl_online_help(''Topic'',''TL_Constant''),else, web([''jar:file:///'',matlabroot,''/help/toolbox/simulink/help.jar!/slref/' lower(get_param(gcbh,'Blocktype')) '.html''], ''-helpbrowser''),end'])
      mask Display: plot([-0.05, 1.05, NaN, -0.05, 1.05],[.01, .01, NaN, .99, .99])
  No step Order Type : Constant  Value=ddv('SAD/Macros/Steps/KU8_NO_STEP_TYPE')  OutDataTypeStr=uint8  mask(TL_Constant){data={'output',{'variable','SAD/Macros/Steps/KU8_NO_STEP_TYPE'},'date',738322.44227276626}}
      settings: CopyFcn=if exist('tl_reset_reviewflag','file')==2,tl_reset_reviewflag(gcbh);end  DeleteFcn=if exist('delete_tlblock','file')==2,delete_tlblock(gcbh);end  NameChangeFcn=if exist('rename_tlblock','file')==2,rename_tlblock(gcbh);end  OpenFcn=if exist('tl_open_blockdlg','file')==2,tl_open_blockdlg(gcbh);else,open_system(gcbh,'parameter');end
      mask Help: eval(['if exist(''tl_online_help'',''file'') == 2, tl_online_help(''Topic'',''TL_Constant''),else, web([''jar:file:///'',matlabroot,''/help/toolbox/simulink/help.jar!/slref/' lower(get_param(gcbh,'Blocktype')) '.html''], ''-helpbrowser''),end'])
      mask Display: plot([-0.05, 1.05, NaN, -0.05, 1.05],[.01, .01, NaN, .99, .99])
  s32RawIncrementValue : Outport  InitialOutput=0
  s32RawFirstOrderValue : Outport  Port=2  InitialOutput=0
  u8RawOrderType : Outport  Port=3  InitialOutput=7
  wires:
  Motor power order shall be reset/1 -> s32RawIncrementValue/1
  Motor power order shall be reset1/1 -> s32RawFirstOrderValue/1
  No step Order Type/1 -> u8RawOrderType/1

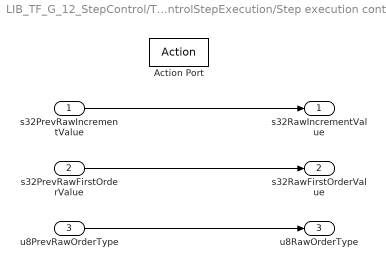
== system LIB_TF_G_12_StepControl/TF_G_12_ControlStepExecution/Step execution continues ==
  s32PrevRawIncrementValue : Inport
  s32PrevRawFirstOrderValue : Inport  Port=2
  u8PrevRawOrderType : Inport  Port=3
  Action Port : ActionPort
  s32RawIncrementValue : Outport  InitialOutput=0
  s32RawFirstOrderValue : Outport  Port=2  InitialOutput=0
  u8RawOrderType : Outport  Port=3  InitialOutput=7
  wires:
  u8PrevRawOrderType/1 -> u8RawOrderType/1
  s32PrevRawIncrementValue/1 -> s32RawIncrementValue/1
  s32PrevRawFirstOrderValue/1 -> s32RawFirstOrderValue/1
